simulink model "htx_amk_eff_estimator_base"  (R2024b)
settings: Solver=FixedStepAuto  StartTime=0.0  StopTime=10.0  FixedStep=0.004  RelTol=1e-3
undefined symbols (not defined in the file): AMKData, AMKData_T100C, AMKData_T120C
settings Model: SimulationMode=accelerator  Creator=lukec  LastModifiedBy=lukec
settings SolverCC: ZeroCrossControl=DisableAll
settings OptimizationCC: DefaultParameterBehavior=Inlined  EnhancedBackFolding=on  PassReuseOutputArgsAs=Individual arguments  ZeroExternalMemoryAtStartup=off  ZeroInternalMemoryAtStartup=off  OptimizeBlockOrder=speed  DifferentSizesBufferReuse=on  OptimizationCustomize=off  EfficientTunableParamExpr=on
settings DebuggingCC: ParameterTunabilityLossMsg=error
settings HardwareCC: ProdBitPerPointer=32  ProdBitPerSizeT=32  ProdBitPerPtrDiffT=32  ProdLargestAtomicInteger=Long  ProdLargestAtomicFloat=Double  ProdWordSize=32  ProdHWDeviceType=ARM Compatible->ARM Cortex-M
settings SFSimCC: MATLABDynamicMemAlloc=off
settings RTWCC: Description=Embedded Coder  SystemTargetFile=ert.tlc  GenCodeOnly=on  PackageGeneratedCodeAndArtifacts=on  TemplateMakefile=ert_default_tmf  Toolchain=CMake  TargetLang=C++
settings CodeAppCC: ForceParamTrailComments=on  IgnoreCustomStorageClasses=off  MaxIdLength=255  OperatorAnnotations=on  SimulinkDataObjDesc=on  SFDataObjDesc=on  InsertBlockDesc=on
settings ERTTargetCC: TargetLangStandard=C++17 (ISO)  GenerateSampleERTMain=on  CodeInterfacePackaging=C++ class  RootIOFormat=Structure reference  ERTCustomFileTemplate=example_file_process.tlc  ArrayContainerType=std::array

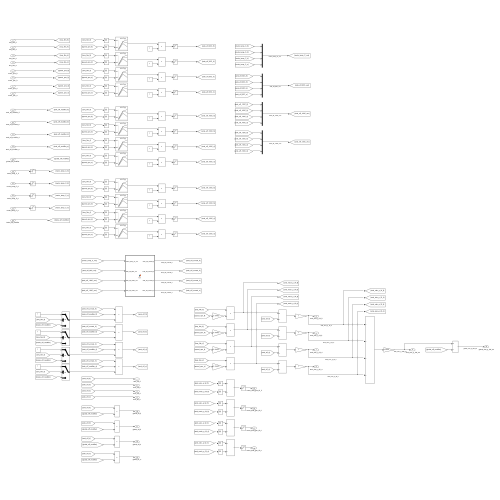
[thumbnail: Simulink's stored preview of the top-level diagram]
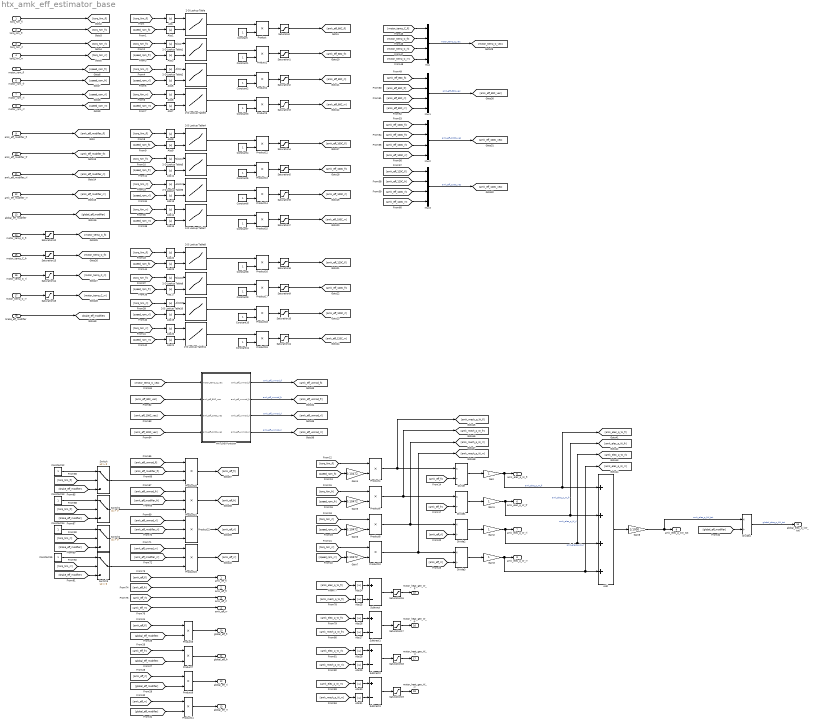
== system htx_amk_eff_estimator_base ==
  torq_Nm_fl : Inport
  torq_Nm_fr : Inport  Port=2
  torq_Nm_rl : Inport  Port=3
  torq_Nm_rr : Inport  Port=4
  motor_rpm_fl : Inport  Port=5
  motor_rpm_fr : Inport  Port=6
  motor_rpm_rl : Inport  Port=7
  motor_rpm_rr : Inport  Port=8
  amk_eff_modifier_fl : Inport  Port=9
  amk_eff_modifier_fr : Inport  Port=10
  amk_eff_modifier_rl : Inport  Port=11
  amk_eff_modifier_rr : Inport  Port=12
  global_eff_modifier : Inport  Port=13
  motor_temp_C_fl : Inport  Port=14
  motor_temp_C_fr : Inport  Port=15
  motor_temp_C_rl : Inport  Port=16
  motor_temp_C_rr : Inport  Port=17
  brake_eff_modifier : Inport  Port=18
  2-D Lookup Table{,1..3} (4 alike) : Lookup_n-D  BreakpointsForDimension1=AMKData.torq_testpoints  BreakpointsForDimension2=AMKData.speed_testpoints  Table=AMKData.eff_zq  InternalRulePriority=Speed  RndMeth=Simplest
      settings: InputPortMap=u0,u1
  2-D Lookup Table{8..11} (4 alike) : Lookup_n-D  BreakpointsForDimension1=AMKData_T120C.torq_testpoints  BreakpointsForDimension2=AMKData_T120C.speed_testpoints  Table=AMKData_T120C.eff_zq  InternalRulePriority=Speed  RndMeth=Simplest
      settings: InputPortMap=u0,u1
  2-D Lookup Table{4..7} (4 alike) : Lookup_n-D  BreakpointsForDimension1=AMKData_T100C.torq_testpoints  BreakpointsForDimension2=AMKData_T100C.speed_testpoints  Table=AMKData_T100C.eff_zq  InternalRulePriority=Speed  RndMeth=Simplest
      settings: InputPortMap=u0,u1
  Abs{,1..31} (32 alike) : Abs  SaturateOnIntegerOverflow=off
  Add : Sum  Inputs=++++
  Constant{,1..15} (16 alike) : Constant
  Divide{,1..4} (5 alike) : Product  Inputs=*/
  Gain{,1..3} (4 alike) : Gain
  Gain{4..7} (4 alike) : Gain  Gain=0.10472
  Gain8 : Gain  Gain=1/1000
  MATLAB Function : MATLAB Function  TreatAsAtomicUnit=on
  Mux{,1..3} (4 alike) : Mux
  Product{,1..19} (20 alike) : Product
  Product{20..23} (4 alike) : Product  Inputs=3
  Saturation{,1..11} (12 alike) : Saturate  UpperLimit=1  LowerLimit=0.6
  Saturation{12..15} (4 alike) : Saturate  UpperLimit=120  LowerLimit=80
  Saturation{16..19} (4 alike) : Saturate  UpperLimit=inf  LowerLimit=0
  Subtract{,1..3} (4 alike) : Sum  Inputs=+-
  Switch{,1..3} (4 alike) : Switch  Criteria=u2 > Threshold  SaturateOnIntegerOverflow=off  InputSameDT=off
  amk_eff_fl : Outport
  amk_eff_fr : Outport  Port=2
  amk_eff_rl : Outport  Port=3
  amk_eff_rr : Outport  Port=4
  amk_elec_p_W_fl : Outport  Port=5
  amk_elec_p_W_fr : Outport  Port=6
  amk_elec_p_W_rl : Outport  Port=7
  amk_elec_p_W_rr : Outport  Port=8
  amk_elec_p_kW_tot : Outport  Port=9
  global_eff_fl : Outport  Port=10
  global_eff_fr : Outport  Port=11
  global_eff_rl : Outport  Port=12
  global_eff_rr : Outport  Port=13
  global_elec_p_kW_tot : Outport  Port=14
  motor_heat_gen_W_fl : Outport  Port=15
  motor_heat_gen_W_fr : Outport  Port=16
  motor_heat_gen_W_rl : Outport  Port=17
  motor_heat_gen_W_rr : Outport  Port=18
  wires:
  [brake_eff_modifier] -> Switch1/3
  Switch2/1 -> Product22/3
  [brake_eff_modifier] -> Switch/3
  Constant14/1 -> Switch2/1
  [brake_eff_modifier] -> Switch2/3
  [torq_Nm_rl] -> Switch2/2
  Constant12/1 -> Switch/1
  Switch3/1 -> Product23/3
  [torq_Nm_rr] -> Abs20/1
  [amk_eff_100C_rr] -> Mux2/4
  [speed_rpm_rr] -> Abs15/1
  Abs16/1 -> 2-D Lookup Table9/1
  Saturation2/1 -> [amk_eff_80C_rl]
  Subtract2/1 -> Saturation18/1
  2-D Lookup Table11/1 -> Product19/1
  Gain2/1 -> [amk_elec_p_W_rl], Add/3, amk_elec_p_W_rl/1  "amk_elec_p_W_rl"
  Saturation7/1 -> [amk_eff_100C_rr]
  Abs17/1 -> 2-D Lookup Table9/2
  Abs18/1 -> 2-D Lookup Table10/1
  Abs19/1 -> 2-D Lookup Table10/2
  Abs21/1 -> 2-D Lookup Table11/2
  Saturation11/1 -> [amk_eff_120C_rr]
  Abs9/1 -> 2-D Lookup Table4/2
  Abs10/1 -> 2-D Lookup Table5/1
  Abs8/1 -> 2-D Lookup Table4/1
  Abs11/1 -> 2-D Lookup Table5/2
  Product/1 -> Saturation/1
  [amk_eff_100C_fl] -> Mux2/1
  [speed_rpm_fr] -> Abs11/1
  motor_rpm_fr/1 -> [speed_rpm_fr]
  [amk_eff_120C_rl] -> Mux3/3
  [torq_Nm_rl] -> Product8/1
  Mux/1 -> [motor_temp_C_vec]  "motor_temp_C_vec"
  [torq_Nm_rr] -> Abs14/1
  [global_eff_modifier] -> Divide4/2
  Constant9/1 -> Product17/2
  [speed_rpm_rr] -> Gain7/1
  Mux3/1 -> [amk_eff_120C_vec]  "amk_eff_120C_vec"
  motor_rpm_rr/1 -> [speed_rpm_rr]
  Product17/1 -> Saturation9/1
  Saturation1/1 -> [amk_eff_80C_fr]
  Constant1/1 -> Product1/2
  Constant6/1 -> Product14/2
  [amk_eff_80C_rr] -> Mux1/4
  Product4/1 -> [amk_mech_p_W_fl], Divide/1
  Gain7/1 -> Product10/2
  Product21/1 -> [amk_eff_fr]
  Abs28/1 -> Subtract2/1
  [amk_eff_120C_fr] -> Mux3/2
  Divide/1 -> Gain/1
  [speed_rpm_fr] -> Abs17/1
  2-D Lookup Table9/1 -> Product17/1
  Subtract/1 -> Saturation16/1
  [amk_eff_rl] -> Divide2/2
  Constant7/1 -> Product15/2
  MATLAB Function/4(amk_eff_unmod_rr) -> [amk_eff_unmod_rr]  "amk_eff_unmod_rr"
  Product3/1 -> Saturation3/1
  Product1/1 -> Saturation1/1
  motor_temp_C_fr/1 -> Saturation13/1
  Divide4/1 -> global_elec_p_kW_tot/1  "global_elec_p_kW_tot"
  [amk_mech_p_W_fl] -> Abs25/1
  [torq_Nm_fl] -> Abs8/1
  Saturation14/1 -> [motor_temp_C_rl]
  Product15/1 -> Saturation7/1
  [amk_eff_fr] -> Product7/1
  [global_eff_modifier] -> Product11/2
  Switch/1 -> Product20/3
  [torq_Nm_fl] -> Switch/2
  Product13/1 -> Saturation5/1
  torq_Nm_rl/1 -> [torq_Nm_rl]
  [amk_eff_modifier_rr] -> Product23/2
  [amk_eff_modifier_fl] -> Product20/2
  [amk_eff_rr] -> Product11/1
  Gain1/1 -> [amk_elec_p_W_fr], Add/2, amk_elec_p_W_fr/1  "amk_elec_p_W_fr"
  Abs24/1 -> Subtract/1
  Add/1 -> Gain8/1
  Abs14/1 -> 2-D Lookup Table7/1
  Gain4/1 -> Product4/2
  [torq_Nm_fr] -> Product6/1
  2-D Lookup Table1/1 -> Product1/1
  [motor_temp_C_fl] -> Mux/1
  Saturation13/1 -> [motor_temp_C_fr]
  Saturation12/1 -> [motor_temp_C_fl]
  [amk_eff_rr] -> Divide3/2
  Divide3/1 -> Gain3/1
  Constant2/1 -> Product2/2
  [amk_eff_unmod_fr] -> Product21/1
  Abs23/1 -> 2-D Lookup Table8/2
  [amk_eff_100C_fr] -> Mux2/2
  Gain6/1 -> Product8/2
  Constant5/1 -> Product13/2
  Saturation19/1 -> motor_heat_gen_W_rr/1
  [speed_rpm_rl] -> Gain6/1
  [amk_eff_unmod_fl] -> Product20/1
  [motor_temp_C_vec] -> MATLAB Function/1(motor_temp_C_vec)
  [amk_eff_120C_fl] -> Mux3/1
  Constant8/1 -> Product16/2
  [motor_temp_C_fr] -> Mux/2
  [motor_temp_C_rr] -> Mux/4
  torq_Nm_rr/1 -> [torq_Nm_rr]
  Saturation4/1 -> [amk_eff_100C_fl]
  [torq_Nm_rl] -> Abs18/1
  [amk_eff_modifier_fr] -> Product21/2
  Gain5/1 -> Product6/2
  [torq_Nm_fl] -> Abs22/1
  [speed_rpm_fl] -> Abs9/1
  [amk_eff_120C_rr] -> Mux3/4
  [torq_Nm_fl] -> Abs/1
  amk_eff_modifier_fr/1 -> [amk_eff_modifier_fr]
  Saturation6/1 -> [amk_eff_100C_rl]
  [amk_eff_rl] -> Product9/1
  [amk_eff_fl] -> amk_eff_fl/1
  Mux2/1 -> [amk_eff_100C_vec]  "amk_eff_100C_vec"
  Abs25/1 -> Subtract/2
  Product19/1 -> Saturation11/1
  Saturation3/1 -> [amk_eff_80C_rr]
  [speed_rpm_rr] -> Abs21/1
  [amk_eff_fr] -> Divide1/2
  [amk_mech_p_W_fr] -> Abs27/1
  [torq_Nm_fr] -> Switch1/2
  [amk_eff_100C_vec] -> MATLAB Function/3(amk_eff_100C_vec)
  amk_eff_modifier_rl/1 -> [amk_eff_modifier_rl]
  Constant11/1 -> Product19/2
  [amk_elec_p_W_rr] -> Abs30/1
  [amk_eff_80C_fl] -> Mux1/1
  Product12/1 -> Saturation4/1
  [amk_eff_fl] -> Product5/1
  Abs26/1 -> Subtract1/1
  [amk_eff_fr] -> amk_eff_fr/1
  [torq_Nm_rl] -> Abs12/1
  [torq_Nm_rr] -> Abs6/1
  MATLAB Function/1(amk_eff_unmod_fl) -> [amk_eff_unmod_fl]  "amk_eff_unmod_fl"
  [speed_rpm_fr] -> Gain5/1
  Constant/1 -> Product/2
  2-D Lookup Table4/1 -> Product12/1
  [motor_temp_C_rl] -> Mux/3
  Product6/1 -> [amk_mech_p_W_fr], Divide1/1
  Product5/1 -> global_eff_fl/1
  Product8/1 -> [amk_mech_p_W_rl], Divide2/1
  [amk_eff_80C_vec] -> MATLAB Function/2(amk_eff_80C_vec)
  global_eff_modifier/1 -> [global_eff_modifier]
  Abs5/1 -> 2-D Lookup Table2/2
  Product2/1 -> Saturation2/1
  Abs27/1 -> Subtract1/2
  [amk_mech_p_W_rr] -> Abs31/1
  Switch1/1 -> Product21/3
  MATLAB Function/3(amk_eff_unmod_rl) -> [amk_eff_unmod_rl]  "amk_eff_unmod_rl"
  [speed_rpm_fl] -> Abs1/1
  Product22/1 -> [amk_eff_rl]
  [amk_eff_rr] -> amk_eff_rr/1
  Saturation10/1 -> [amk_eff_120C_rl]
  [speed_rpm_rr] -> Abs7/1
  Gain/1 -> Add/1, [amk_elec_p_W_fl], amk_elec_p_W_fl/1  "amk_elec_p_W_fl"
  [amk_elec_p_W_fl] -> Abs24/1
  Product16/1 -> Saturation8/1
  Subtract1/1 -> Saturation17/1
  Product23/1 -> [amk_eff_rr]
  [speed_rpm_fr] -> Abs3/1
  2-D Lookup Table5/1 -> Product13/1
  Product20/1 -> [amk_eff_fl]
  [amk_mech_p_W_rl] -> Abs29/1
  [amk_eff_unmod_rl] -> Product22/1
  [speed_rpm_rl] -> Abs5/1
  Abs/1 -> 2-D Lookup Table/1
  Abs12/1 -> 2-D Lookup Table6/1
  2-D Lookup Table3/1 -> Product3/1
  Abs4/1 -> 2-D Lookup Table2/1
  [speed_rpm_rl] -> Abs13/1
  Abs6/1 -> 2-D Lookup Table3/1
  [global_eff_modifier] -> Product5/2
  2-D Lookup Table8/1 -> Product16/1
  2-D Lookup Table6/1 -> Product14/1
  Abs1/1 -> 2-D Lookup Table/2
  2-D Lookup Table2/1 -> Product2/1
  Abs2/1 -> 2-D Lookup Table1/1
  Product10/1 -> [amk_mech_p_W_rr], Divide3/1
  Constant13/1 -> Switch1/1
  Saturation8/1 -> [amk_eff_120C_fl]
  Abs3/1 -> 2-D Lookup Table1/2
  Gain8/1 -> Divide4/1, amk_elec_p_kW_tot/1  "amk_elec_p_kW_tot"
  [global_eff_modifier] -> Product7/2
  [speed_rpm_rl] -> Abs19/1
  Constant4/1 -> Product12/2
  [amk_eff_80C_rl] -> Mux1/3
  [global_eff_modifier] -> Product9/2
  [amk_eff_unmod_rr] -> Product23/1
  [amk_elec_p_W_rl] -> Abs28/1
  motor_temp_C_fl/1 -> Saturation12/1
  Saturation/1 -> [amk_eff_80C_fl]
  Abs20/1 -> 2-D Lookup Table11/1
  motor_temp_C_rl/1 -> Saturation14/1
  motor_rpm_rl/1 -> [speed_rpm_rl]
  amk_eff_modifier_rr/1 -> [amk_eff_modifier_rr]
  [amk_eff_120C_vec] -> MATLAB Function/4(amk_eff_120C_vec)
  amk_eff_modifier_fl/1 -> [amk_eff_modifier_fl]
  Product7/1 -> global_eff_fr/1
  Abs15/1 -> 2-D Lookup Table7/2
  [amk_elec_p_W_fr] -> Abs26/1
  Mux1/1 -> [amk_eff_80C_vec]  "amk_eff_80C_vec"
  [brake_eff_modifier] -> Switch3/3
  [amk_eff_80C_fr] -> Mux1/2
  Product14/1 -> Saturation6/1
  Abs22/1 -> 2-D Lookup Table8/1
  [speed_rpm_fl] -> Gain4/1
  motor_temp_C_rr/1 -> Saturation15/1
  MATLAB Function/2(amk_eff_unmod_fr) -> [amk_eff_unmod_fr]  "amk_eff_unmod_fr"
  Abs30/1 -> Subtract3/1
  Abs13/1 -> 2-D Lookup Table6/2
  2-D Lookup Table10/1 -> Product18/1
  [amk_eff_100C_rl] -> Mux2/3
  [torq_Nm_fr] -> Abs2/1
  [speed_rpm_fl] -> Abs23/1
  Divide1/1 -> Gain1/1
  Subtract3/1 -> Saturation19/1
  Saturation5/1 -> [amk_eff_100C_fr]
  [amk_eff_rl] -> amk_eff_rl/1
  motor_rpm_fl/1 -> [speed_rpm_fl]
  torq_Nm_fr/1 -> [torq_Nm_fr]
  Saturation18/1 -> motor_heat_gen_W_rl/1
  [torq_Nm_rr] -> Switch3/2
  2-D Lookup Table/1 -> Product/1
  [torq_Nm_fl] -> Product4/1
  Product11/1 -> global_eff_rr/1
  Saturation16/1 -> motor_heat_gen_W_fl/1
  Saturation9/1 -> [amk_eff_120C_fr]
  Gain3/1 -> [amk_elec_p_W_rr], Add/4, amk_elec_p_W_rr/1  "amk_elec_p_W_rr"
  [torq_Nm_rr] -> Product10/1
  Abs7/1 -> 2-D Lookup Table3/2
  brake_eff_modifier/1 -> [brake_eff_modifier]
  Divide2/1 -> Gain2/1
  [torq_Nm_rl] -> Abs4/1
  [torq_Nm_fr] -> Abs10/1
  Saturation15/1 -> [motor_temp_C_rr]
  Constant3/1 -> Product3/2
  torq_Nm_fl/1 -> [torq_Nm_fl]
  Constant10/1 -> Product18/2
  Abs29/1 -> Subtract2/2
  Saturation17/1 -> motor_heat_gen_W_fr/1
  2-D Lookup Table7/1 -> Product15/1
  [torq_Nm_fr] -> Abs16/1
  Constant15/1 -> Switch3/1
  Abs31/1 -> Subtract3/2
  Product9/1 -> global_eff_rl/1
  Product18/1 -> Saturation10/1
  [amk_eff_fl] -> Divide/2
  [amk_eff_modifier_rl] -> Product22/2

== matlab function htx_amk_eff_estimator_base/MATLAB Function ==
  data: motor_temp_C_vec input; amk_eff_unmod_fl output; amk_eff_80C_vec input; amk_eff_100C_vec input; amk_eff_120C_vec input; amk_eff_unmod_fr output; amk_eff_unmod_rl output; amk_eff_unmod_rr output
function [amk_eff_unmod_fl, amk_eff_unmod_fr, amk_eff_unmod_rl, amk_eff_unmod_rr]  = fcn(motor_temp_C_vec, amk_eff_80C_vec, amk_eff_100C_vec, amk_eff_120C_vec)

amk_eff_vec = [1; 1; 1; 1];

for i = 1:4
    temp_C = motor_temp_C_vec(i);
    eff_80C = amk_eff_80C_vec(i);
    eff_100C = amk_eff_100C_vec(i);
    eff_120C = amk_eff_120C_vec(i);

    amk_eff_vec(i) = interp1([80, 100, 120], [eff_80C, eff_100C, eff_120C], temp_C);
end

amk_eff_unmod_fl = amk_eff_vec(1);
amk_eff_unmod_fr = amk_eff_vec(2);
amk_eff_unmod_rl = amk_eff_vec(3);
amk_eff_unmod_rr = amk_eff_vec(4);
